simulink model "TFMODEL"  (R2015a)
settings: Solver=ode45  StartTime=0.0  StopTime=1  RelTol=1e-3
settings Model: Creator=John  LastModifiedBy=John

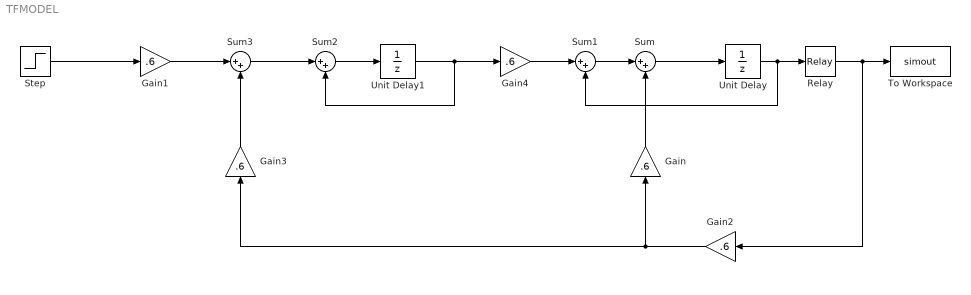
== system TFMODEL ==
  Gain{,1..4} (5 alike) : Gain  Gain=.6
  Relay : Relay
  Step : Step  SampleTime=0
  Sum{,1..3} (4 alike) : Sum  Inputs=|++
  To Workspace : ToWorkspace  VariableName=simout  SaveFormat=Timeseries  SampleTime=-1
  Unit Delay : UnitDelay  SampleTime=-1
  Unit Delay1 : UnitDelay  SampleTime=-1
  wires:
  Step/1 -> Gain1/1
  Gain1/1 -> Sum3/1
  Sum3/1 -> Sum2/1
  Sum2/1 -> Unit Delay1/1
  Gain3/1 -> Sum3/2
  Unit Delay1/1 -> Gain4/1, Sum2/2
  Sum1/1 -> Sum/1
  Gain/1 -> Sum/2
  Sum/1 -> Unit Delay/1
  Gain2/1 -> Gain3/1, Gain/1
  Unit Delay/1 -> Sum1/2, Relay/1
  Relay/1 -> Gain2/1, To Workspace/1
  Gain4/1 -> Sum1/1
